simulink subsystem "Motores"  (R2023b)
settings: Solver=VariableStepAuto  StartTime=0.0  StopTime=10.0  RelTol=1e-3
libraries: arduinolib x6, simulink x2
settings Model: Creator=johan  LastModifiedBy=Carlos

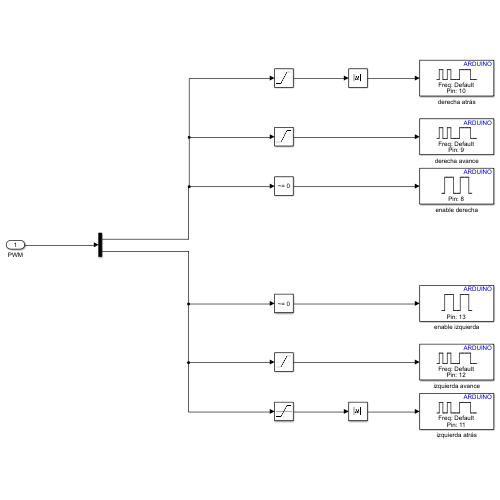
[thumbnail: Simulink's stored preview of the top-level diagram]
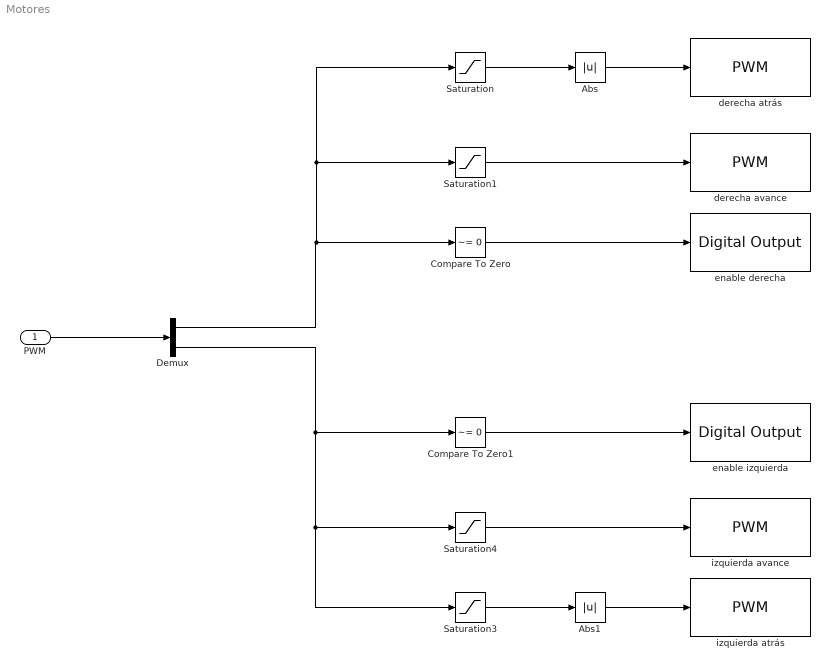
== system Motores ==
  PWM : Inport  OutDataTypeStr=int16
  Abs : Abs  SaturateOnIntegerOverflow=off
  Abs1 : Abs  OutDataTypeStr=int16  SaturateOnIntegerOverflow=off
  Compare To Zero : simulink/Logic and Bit Operations/Compare To Zero  relop=~=  OutDataTypeStr=boolean
  Compare To Zero1 : simulink/Logic and Bit Operations/Compare To Zero  relop=~=  OutDataTypeStr=boolean
  Demux : Demux  Outputs=2
  Saturation : Saturate  UpperLimit=0  LowerLimit=-255
  Saturation1 : Saturate  UpperLimit=255  LowerLimit=0
  Saturation3 : Saturate  UpperLimit=255  LowerLimit=0
  Saturation4 : Saturate  UpperLimit=0  LowerLimit=-255
  derecha atrás : arduinolib/PWM  pinNumber=10  frequencyType=Default  desiredFrequency=490.2  achievableFrequency=490.2
  derecha avance : arduinolib/PWM  pinNumber=9  frequencyType=Default  desiredFrequency=490.2  achievableFrequency=490.2
  enable derecha : arduinolib/Digital Output  pinNumber=8  Direction=output  blockPlatform=arduino
  enable izquierda : arduinolib/Digital Output  pinNumber=13  Direction=output  blockPlatform=arduino
  izquierda atrás : arduinolib/PWM  pinNumber=11  frequencyType=Default  desiredFrequency=490.2  achievableFrequency=490.2
  izquierda avance : arduinolib/PWM  pinNumber=12  frequencyType=Default  desiredFrequency=490.2  achievableFrequency=490.2
  wires:
  PWM/1 -> Demux/1
  Compare To Zero1/1 -> enable izquierda/1
  Saturation4/1 -> izquierda avance/1
  Saturation3/1 -> Abs1/1
  Abs1/1 -> izquierda atrás/1
  Compare To Zero/1 -> enable derecha/1
  Saturation1/1 -> derecha avance/1
  Abs/1 -> derecha atrás/1
  Saturation/1 -> Abs/1
  Demux/1 -> Saturation/1, Saturation1/1, Compare To Zero/1
  Demux/2 -> Saturation3/1, Saturation4/1, Compare To Zero1/1
